simulink model "PID_Cntrl"  (R2020b)
settings: Solver=VariableStepAuto  StartTime=0.0  StopTime=0.2  RelTol=1e-3
undefined symbols (not defined in the file or in its folder): Kd, Ki, Kp
settings Model: DataDictionary=MotorPositionCntrl_data.sldd  Creator=BIDITA PAUL  LastModifiedBy=BIDITA PAUL
settings DataIOCC: SaveOutput=off  SaveTime=off

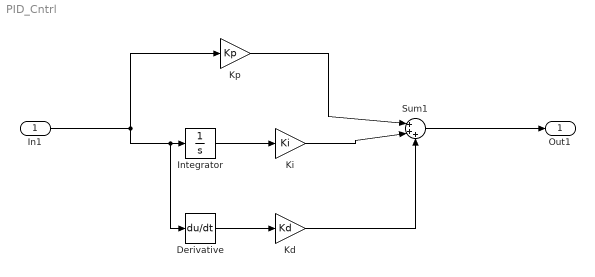
== system PID_Cntrl ==
  In1 : Inport  OutDataTypeStr=double  PortDimensions=1  SampleTime=0
  Derivative : Derivative
  Integrator : Integrator
  Kd : Gain  Gain=Kd
  Ki : Gain  Gain=Ki
  Kp : Gain  Gain=Kp
  Sum1 : Sum  Inputs=|+++
  Out1 : Outport  OutDataTypeStr=double  PortDimensions=1  SampleTime=0
  wires:
  Derivative/1 -> Kd/1
  Kp/1 -> Sum1/1
  Ki/1 -> Sum1/2
  Sum1/1 -> Out1/1
  In1/1 -> Kp/1, Integrator/1, Derivative/1
  Kd/1 -> Sum1/3
  Integrator/1 -> Ki/1
